simulink model "hybrid_lht_accumulator_backup"  (R2019b)
settings: Solver=FixedStepDiscrete  StartTime=0.0  StopTime=inf  FixedStep=1/bt.frequency  RelTol=1e-3
InitFcn:
  | ht_hybrid_setup;
StopFcn:
  | ht_hybrid_compare;
undefined symbols (not defined in the file or in its folder): bt, height, Ntheta, nTheta, width
libraries: hdlsllib x52, simulink x24, visionhdlutilities x2, dspsrcs4 x1, visionhdlio x1, lib_hybrid_ht_kernel x1, visionsources x1
(part 1 of 5)
settings Model: SimulationMode=accelerator  Creator=rgb11127  LastModifiedBy=rgb11127
settings DataIOCC: SaveOutput=off  SaveTime=off  ReturnWorkspaceOutputs=off

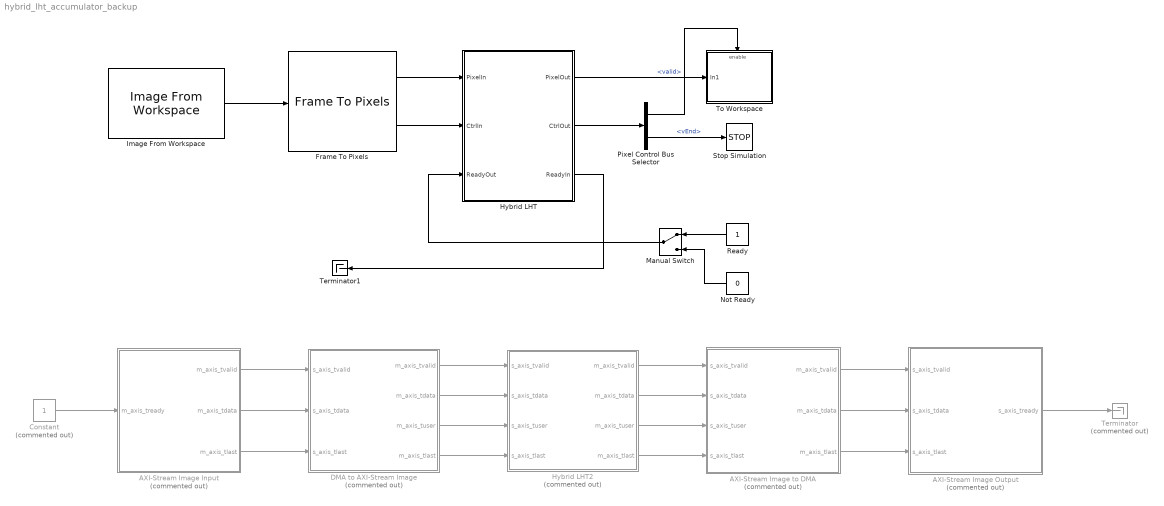
== system hybrid_lht_accumulator_backup ==
  AXI-Stream Image Input : Subsystem  Commented=on  mask{image=bt.inputImage, clk=1/150e6}
      mask prompts: image "Input Image:"; clk "Clock Rate:"
      mask init:
      | [height, width] = size(image);
      mask DialogControl DescGroupVar Prompt: AXI-Stream Image Input
      mask DialogControl DescTextVar Prompt: This block simulates an AXI-Stream image input for interfacing to a hardware accelerator or IP Core.
      mask DialogControl ParameterGroupVar Prompt: Main
  AXI-Stream Image Output : Subsystem  Commented=on  mask{height=bt.nRho, width=bt.nTheta, clk=1/150e6, d=0}
      mask prompts: height "Image Height:"; width "Image Width:"; clk "Clock Rate:"; d "Frame Capture Number"
      mask DialogControl DescGroupVar Prompt: AXI-Stream Image Output
      mask DialogControl DescTextVar Prompt: Image output using the AXI-Stream interface. Simulates an AXI DMA write channel.
      mask DialogControl ParameterGroupVar Prompt: Main
  AXI-Stream Image to DMA : Subsystem  Commented=on  mask{height=bt.nRho, width=bt.nTheta}
      mask prompts: height "Image Height"; width "Image Width"
      mask DialogControl DescGroupVar Prompt: AXI-Stream Image to DMA
      mask DialogControl DescTextVar Prompt: Converts from the AXI-Stream video standard to AXI-Stream DMA packet.
      mask DialogControl Container2 Prompt: Main
  Constant : Constant  Commented=on  OutDataTypeStr=boolean  SampleTime=-1
  DMA to AXI-Stream Image : Subsystem  Commented=on  mask{height=bt.height, width=bt.width}
      mask prompts: height "Image Height:"; width "Image Width:"
      mask DialogControl DescGroupVar Prompt: DMA to AXI-Stream Image
      mask DialogControl DescTextVar Prompt: Converts an DMA AXI-Stream packet to the AXI-Stream video standard.
      mask DialogControl Container2 Prompt: Main
  Frame To Pixels : visionhdlio/Frame To Pixels  NumComponents=1  NumPixels=1  VideoFormat=Custom  ActivePixelsPerLine=bt.width  ActiveVideoLines=bt.height  TotalPixelsPerLine=bt.widthpad  TotalVideoLines=bt.heightpad  StartingActiveLine=bt.activeline  FrontPorch=bt.frontporch  SampleTime=0
      settings: SourceProductName=Vision HDL Toolbox  SourceProductBaseCode=VT
  Hybrid LHT : Subsystem  TreatAsAtomicUnit=on
  Hybrid LHT2 : Subsystem  Commented=on
  Image From Workspace : visionsources/Image From Workspace  Tag=vipblks_nd  ImageValue=bt.inputImage  Ts=1/bt.fps  imagePorts=One multidimensional signal  OutPortLabels=R|G|B  ImageDataType=Inherit from 'Value'  Signed=on  WordLength=16  sdImageDataType=sfix(16)  FractionLengthMode=User-defined  FractionLength=15
      settings: SourceProductName=Computer Vision Toolbox  SourceProductBaseCode=VP
  Manual Switch : ManualSwitch
  Not Ready : Constant  Value=0  OutDataTypeStr=boolean  SampleTime=-1
  Pixel Control Bus Selector : BusSelector  OutputSignals=valid,vEnd
  Ready : Constant  OutDataTypeStr=boolean  SampleTime=-1
  Stop Simulation : Stop
  Terminator : Terminator  Commented=on
  Terminator1 : Terminator
  To Workspace : Subsystem  TreatAsAtomicUnit=on
  wires:
  Constant/1 -> AXI-Stream Image Input/1(m_axis_tready)
  AXI-Stream Image Input/1(m_axis_tvalid) -> DMA to AXI-Stream Image/1(s_axis_tvalid)
  AXI-Stream Image Input/2(m_axis_tdata) -> DMA to AXI-Stream Image/2(s_axis_tdata)
  AXI-Stream Image Input/3(m_axis_tlast) -> DMA to AXI-Stream Image/3(s_axis_tlast)
  DMA to AXI-Stream Image/1(m_axis_tvalid) -> Hybrid LHT2/1(s_axis_tvalid)
  DMA to AXI-Stream Image/2(m_axis_tdata) -> Hybrid LHT2/2(s_axis_tdata)
  DMA to AXI-Stream Image/3(m_axis_tuser) -> Hybrid LHT2/3(s_axis_tuser)
  DMA to AXI-Stream Image/4(m_axis_tlast) -> Hybrid LHT2/4(s_axis_tlast)
  AXI-Stream Image Output/1(s_axis_tready) -> Terminator/1
  AXI-Stream Image to DMA/3(m_axis_tlast) -> AXI-Stream Image Output/3(s_axis_tlast)
  AXI-Stream Image to DMA/2(m_axis_tdata) -> AXI-Stream Image Output/2(s_axis_tdata)
  AXI-Stream Image to DMA/1(m_axis_tvalid) -> AXI-Stream Image Output/1(s_axis_tvalid)
  Hybrid LHT2/4(m_axis_tlast) -> AXI-Stream Image to DMA/4(s_axis_tlast)
  Hybrid LHT2/3(m_axis_tuser) -> AXI-Stream Image to DMA/3(s_axis_tuser)
  Hybrid LHT2/2(m_axis_tdata) -> AXI-Stream Image to DMA/2(s_axis_tdata)
  Hybrid LHT2/1(m_axis_tvalid) -> AXI-Stream Image to DMA/1(s_axis_tvalid)
  Not Ready/1 -> Manual Switch/2
  Manual Switch/1 -> Hybrid LHT/3(ReadyOut)
  Ready/1 -> Manual Switch/1
  Hybrid LHT/3(ReadyIn) -> Terminator1/1
  Frame To Pixels/2 -> Hybrid LHT/2(CtrlIn)
  Frame To Pixels/1 -> Hybrid LHT/1(PixelIn)
  Hybrid LHT/2(CtrlOut) -> Pixel Control Bus Selector/1
  Hybrid LHT/1(PixelOut) -> To Workspace/1(In1)
  Pixel Control Bus Selector/1 -> To Workspace/Enable  "<valid>"
  Image From Workspace/1 -> Frame To Pixels/1
  Pixel Control Bus Selector/2 -> Stop Simulation/1  "<vEnd>"

== system hybrid_lht_accumulator_backup/AXI-Stream Image Input ==
  m_axis_tready : Inport
  Compare To Constant : simulink/Logic and Bit Operations/Compare To Constant  relop===  const=height*width-1  OutDataTypeStr=boolean
  HDL Counter : hdlsllib/Sources/HDL Counter  CountType=Count limited  CountInit=0  CountStep=1  CountMax=width*height-1  CountFromType=Initial value  CountFrom=0  CountResetPort=off  CountLoadPort=off  CountEnbPort=on  CountDirPort=off  CountDataType=Unsigned  CountWordLen=ceil(log2(width*height))  CountFracLen=0  CountSampTime=1
      settings: SourceProductName=Simulink
  Master AXI-Stream FIFO : Subsystem  mask{depth=32}
      mask prompts: depth "FIFO Depth:"
      mask DialogControl DescGroupVar Prompt: Master AXI-Stream FIFO
      mask DialogControl DescTextVar Prompt: A custom AXI-Stream FIFO for interfacing to write channel AXI DMAs.
      mask DialogControl ParameterGroupVar Prompt: Main
  Synchronous Image Source : Subsystem
  m_axis_tvalid : Outport
  m_axis_tdata : Outport  Port=2
  m_axis_tlast : Outport  Port=3
  wires:
  Master AXI-Stream FIFO/2(m_axis_tdata) -> m_axis_tdata/1
  Master AXI-Stream FIFO/3(m_axis_tlast) -> m_axis_tlast/1
  m_axis_tready/1 -> Master AXI-Stream FIFO/4(m_axis_tready)
  Master AXI-Stream FIFO/4(s_axis_tready) -> HDL Counter/1, Master AXI-Stream FIFO/1(s_axis_tvalid), Synchronous Image Source/Enable
  Compare To Constant/1 -> Master AXI-Stream FIFO/3(s_axis_tlast)
  Master AXI-Stream FIFO/1(m_axis_tvalid) -> m_axis_tvalid/1
  HDL Counter/1 -> Compare To Constant/1
  Synchronous Image Source/1(Pixel) -> Master AXI-Stream FIFO/2(s_axis_tdata)

== system hybrid_lht_accumulator_backup/AXI-Stream Image Output ==
  s_axis_tvalid : Inport
  s_axis_tdata : Inport  Port=2
  s_axis_tlast : Inport  Port=3
  AND1 : Logic  IconShape=distinctive  AllPortsSameDT=off  OutDataTypeStr=boolean
  Compare To Constant4 : simulink/Logic and Bit Operations/Compare To Constant  relop===  const=(height)*width-1  OutDataTypeStr=boolean
  Constant : Constant  OutDataTypeStr=boolean  SampleTime=-1
  Delay2 : Delay  DelayLength=d  ShowEnablePort=on
      settings: InputPortMap=u0,e6
  Pixel to Workspace : Subsystem
  Stop Simulation1 : Stop
  Terminator : Terminator
  Total Samples Counter : hdlsllib/Sources/HDL Counter  CountType=Count limited  CountInit=0  CountStep=1  CountMax=(height)*width-1  CountFromType=Initial value  CountFrom=0  CountResetPort=off  CountLoadPort=off  CountEnbPort=on  CountDirPort=off  CountDataType=Unsigned  CountWordLen=ceil(log2((height)*width+1))  CountFracLen=0  CountSampTime=1
      settings: SourceProductName=Simulink
  s_axis_tready : Outport  VectorParamsAs1DForOutWhenUnconnected=off
  wires:
  Constant/1 -> s_axis_tready/1, AND1/2
  s_axis_tlast/1 -> Terminator/1
  Delay2/1 -> Stop Simulation1/1
  Compare To Constant4/1 -> Delay2/1, Delay2/2
  Total Samples Counter/1 -> Compare To Constant4/1
  AND1/1 -> Pixel to Workspace/Enable, Total Samples Counter/1
  s_axis_tvalid/1 -> AND1/1
  s_axis_tdata/1 -> Pixel to Workspace/1(Pixel In)

== system hybrid_lht_accumulator_backup/AXI-Stream Image to DMA ==
  s_axis_tvalid : Inport
  s_axis_tdata : Inport  Port=2
  s_axis_tuser : Inport  Port=3
  s_axis_tlast : Inport  Port=4
  AND : Logic  IconShape=distinctive  AllPortsSameDT=off  OutDataTypeStr=boolean
  Compare To Constant : simulink/Logic and Bit Operations/Compare To Constant  relop===  const=height*width-1  OutDataTypeStr=boolean
  Data Type Conversion : DataTypeConversion  OutDataTypeStr=uint32
  Output Counter : hdlsllib/Sources/HDL Counter  CountType=Count limited  CountInit=0  CountStep=1  CountMax=height*width-1  CountFromType=Initial value  CountFrom=0  CountResetPort=off  CountLoadPort=off  CountEnbPort=on  CountDirPort=off  CountDataType=Unsigned  CountWordLen=ceil(log2(height*width))  CountFracLen=0  CountSampTime=1
      settings: SourceProductName=Simulink
  Terminator : Terminator
  Terminator1 : Terminator
  m_axis_tvalid : Outport
  m_axis_tdata : Outport  Port=2
  m_axis_tlast : Outport  Port=3
  wires:
  Data Type Conversion/1 -> m_axis_tdata/1
  s_axis_tdata/1 -> Data Type Conversion/1
  s_axis_tvalid/1 -> AND/2, m_axis_tvalid/1, Output Counter/1
  s_axis_tlast/1 -> Terminator/1
  s_axis_tuser/1 -> Terminator1/1
  Output Counter/1 -> Compare To Constant/1
  Compare To Constant/1 -> AND/1
  AND/1 -> m_axis_tlast/1

== system hybrid_lht_accumulator_backup/DMA to AXI-Stream Image ==
  s_axis_tvalid : Inport
  s_axis_tdata : Inport  Port=2
  s_axis_tlast : Inport  Port=3
  AND : Logic  IconShape=distinctive  AllPortsSameDT=off  OutDataTypeStr=boolean
  AND1 : Logic  IconShape=distinctive  AllPortsSameDT=off  OutDataTypeStr=boolean
  AND2 : Logic  IconShape=distinctive  AllPortsSameDT=off  OutDataTypeStr=boolean
  Compare To Constant : simulink/Logic and Bit Operations/Compare To Constant  relop===  const=width-1  OutDataTypeStr=boolean
  Compare To Zero : simulink/Logic and Bit Operations/Compare To Zero  relop===  OutDataTypeStr=boolean
  Compare To Zero1 : simulink/Logic and Bit Operations/Compare To Zero  relop===  OutDataTypeStr=boolean
  Terminator : Terminator
  X Counter : hdlsllib/Sources/HDL Counter  CountType=Count limited  CountInit=0  CountStep=1  CountMax=width-1  CountFromType=Initial value  CountFrom=0  CountResetPort=off  CountLoadPort=off  CountEnbPort=on  CountDirPort=off  CountDataType=Unsigned  CountWordLen=ceil(log2(width))  CountFracLen=0  CountSampTime=1
      settings: SourceProductName=Simulink
  Y Counter : hdlsllib/Sources/HDL Counter  CountType=Count limited  CountInit=0  CountStep=1  CountMax=height-1  CountFromType=Initial value  CountFrom=0  CountResetPort=off  CountLoadPort=off  CountEnbPort=on  CountDirPort=off  CountDataType=Unsigned  CountWordLen=ceil(log2(height))  CountFracLen=0  CountSampTime=1
      settings: SourceProductName=Simulink
  m_axis_tvalid : Outport
  m_axis_tdata : Outport  Port=2
  m_axis_tuser : Outport  Port=3
  m_axis_tlast : Outport  Port=4
  wires:
  AND2/1 -> m_axis_tlast/1
  Compare To Constant/1 -> Y Counter/1, AND2/2
  AND1/1 -> m_axis_tuser/1
  AND/1 -> AND1/2
  s_axis_tlast/1 -> Terminator/1
  Compare To Zero/1 -> AND/2
  Compare To Zero1/1 -> AND/1
  Y Counter/1 -> Compare To Zero/1
  X Counter/1 -> Compare To Constant/1, Compare To Zero1/1
  s_axis_tvalid/1 -> m_axis_tvalid/1, AND1/1, AND2/1, X Counter/1
  s_axis_tdata/1 -> m_axis_tdata/1

== system hybrid_lht_accumulator_backup/Hybrid LHT ==
  PixelIn : Inport
  CtrlIn : Inport  Port=2
  ReadyOut : Inport  Port=3
  Constant : Constant  Value=60  OutDataTypeStr=uint32  SampleTime=-1
  FIFO Subsystem : Subsystem
  Hybrid LHT Accumulator : Subsystem  AncestorBlock=lib_hybrid_ht_accumulator/Hybrid LHT Accumulator  VariantControl=Basic  mask{w=bt.width, h=bt.height, theta=bt.theta, mode=Parameter Space Readout}
      mask prompts: w "Image Width:"; h "Image Height:"; theta "Orientations:"; mode "Architecture:"
      mask init:
      | % Get parameters
      | maxRho = ceil(sqrt((h/2)^2+(w/2)^2));
      | Nrho = maxRho*2;
      | [~, Ntheta] = size(theta);
      | 
      | % Set correct variants
      | 
      | blk_gen = [gcb, '/Simple Hough Accumulator/Flag Generator'];
      | blk_sep = [gcb, '/Simple Hough Accumulator/Separate Bits'];
      | blk_keep = [gcb, '/Simple Hough Accumulator/Keep Flag'];
      | blk_out = [gcb, '/Output Generation'];
      | 
      | oldVariant = get_param(blk_gen, 'OverrideUsingVariant');
      | 
      | switch get_param(gcb, 'mode')
      |     case 'Video Backprojection'
      |         newVariant = 'Backprojection';
      |         voteWL = ceil(log2(2*maxRho))+1;
      |         videomode = 1;
      |     case 'Parameter Space Readout'
      |         newVariant = 'Passthrough';
      |         voteWL = ceil(log2(2*maxRho));
      |         videomode = 0;
      |     otherwise
      |         newVariant = 'Passthrough';
      |         voteWL = ceil(log2(2*maxRho));
      |         videomode = 0;
      | end
      | 
      | if ~strcmp(oldVariant, newVariant)
      |     set_param(blk_gen, 'OverrideUsingVariant', newVariant);
      |     set_param(blk_sep, 'OverrideUsingVariant', newVariant);
      |     set_param(blk_keep, 'OverrideUsingVariant', newVariant);
      |     set_param(blk_out, 'OverrideUsingVariant', newVariant);
      | end
      mask TypeOptions mode: Video Backprojection | Parameter Space Readout
      mask DialogControl DescGroupVar Prompt: Parallel Hough Accumulator
      mask DialogControl DescTextVar Prompt: The Parallel Hough Accumulator implements a low-latency circuit for storing the Hough Parameter Space. If the mode input is set to '1', the architecture will draw lines using backpropagation. If mode is set to '0', the HPS is output on the HPS and CtrlOut ports.
      mask DialogControl Container2 Prompt: Image Parameters
      mask DialogControl Container3 Prompt: Accumulator Implementation
  Hybrid LHT Kernel : lib_hybrid_ht_kernel/Hybrid LHT Kernel  w=bt.width  h=bt.height  theta=bt.theta
  NOT : Logic  Operator=NOT  IconShape=distinctive  AllPortsSameDT=off  OutDataTypeStr=boolean
  PixelOut : Outport  VectorParamsAs1DForOutWhenUnconnected=off
  CtrlOut : Outport  Port=2  VectorParamsAs1DForOutWhenUnconnected=off
  ReadyIn : Outport  Port=3  VectorParamsAs1DForOutWhenUnconnected=off
  wires:
  NOT/1 -> ReadyIn/1
  ReadyOut/1 -> Hybrid LHT Accumulator/6(Ready)
  FIFO Subsystem/3(ReadyIn) -> NOT/1
  Hybrid LHT Accumulator/2(CtrlOut) -> CtrlOut/1
  PixelIn/1 -> FIFO Subsystem/1(PixelIn)
  CtrlIn/1 -> FIFO Subsystem/2(CtrlIn)
  Hybrid LHT Kernel/2 -> Hybrid LHT Accumulator/3(Rho)
  Hybrid LHT Kernel/3 -> Hybrid LHT Accumulator/4(Shift)
  FIFO Subsystem/2(CtrlOut) -> Hybrid LHT Kernel/2
  Hybrid LHT Kernel/5 -> FIFO Subsystem/3(POP)
  Hybrid LHT Kernel/1 -> Hybrid LHT Accumulator/2(vEdge)
  Constant/1 -> Hybrid LHT Accumulator/1(Threshold)
  FIFO Subsystem/1(PixelOut) -> Hybrid LHT Kernel/1
  Hybrid LHT Kernel/4 -> Hybrid LHT Accumulator/5(CtrlIn)
  Hybrid LHT Accumulator/1(Pixel) -> PixelOut/1

== system hybrid_lht_accumulator_backup/Hybrid LHT2 ==
  s_axis_tvalid : Inport
  s_axis_tdata : Inport  Port=2
  s_axis_tuser : Inport  Port=3
  s_axis_tlast : Inport  Port=4
  Constant : Constant  Commented=on  OutDataTypeStr=uint8  SampleTime=-1
  Constant1 : Constant  Commented=on  OutDataTypeStr=boolean  SampleTime=-1
  Hybrid LHT Accumulator : Subsystem  mask{height=bt.height, width=bt.width, theta=bt.theta}
      mask prompts: height "Image Height:"; width "Image Width:"; theta "Orientations:"
      mask init:
      | maxRho = ceil(sqrt((height/2)^2+(width/2)^2));
      | nRho = maxRho*2;
      | [~, nTheta] = size(theta);
      | 
      | voteWL = ceil(log2(2*maxRho));
      mask DialogControl ParameterGroupVar Prompt: Main
  Hybrid LHT Accumulator2 : Subsystem  Commented=on  VariantControl=Basic  mask{w=bt.width, h=bt.height, theta=bt.theta, mode=Parameter Space Readout}
      mask prompts: w "Image Width:"; h "Image Height:"; theta "Orientations:"; mode "Architecture:"
      mask init: same as hybrid_lht_accumulator_backup/Hybrid LHT/Hybrid LHT Accumulator
      mask TypeOptions mode: Video Backprojection | Parameter Space Readout
      mask DialogControl DescGroupVar Prompt: Parallel Hough Accumulator
      mask DialogControl DescTextVar Prompt: The Parallel Hough Accumulator implements a low-latency circuit for storing the Hough Parameter Space. If the mode input is set to '1', the architecture will draw lines using backpropagation. If mode is set to '0', the HPS is output on the HPS and CtrlOut ports.
      mask DialogControl Container2 Prompt: Image Parameters
      mask DialogControl Container3 Prompt: Accumulator Implementation
  Hybrid LHT Kernel : Subsystem  mask{height=bt.height, width=bt.width, theta=bt.theta}
      mask prompts: height "Image Height:"; width "Image Width:"; theta "Orientations:"
      mask init:
      | % Get number of orientations to operate across
      | [~, nTheta] = size(theta);
      | 
      | % Get discretisation step of theta
      | if nTheta > 1
      |     dTheta = theta(end) - theta(end-1);
      | else
      |     dTheta = 1;
      | end
      | 
      | % Get the maximum magnitude of displacement
      | maxRho = ceil(sqrt((height/2)^2+(width/2)^2));
      | 
      | % Get the number of bits required to vote correctly
      | voteWL = ceil(log2(maxRho*2));
      | 
      | % Get the number of division possible
      | if nTheta < floor(36/voteWL)
      |     L = nTheta;
      | else
      |     L = floor(36/voteWL);
      | end
      | 
      | % Set lambda, the number of orientations to operate across per gradient
      | % orientation given
      | lambda = floor(nTheta/(2*L));
      | 
      | % Determine if the number of orientations is odd. This will prevent over
      | % use of the parameter space.
      | if lambda == 0
      |     subflag = 0;
      | else
      |     subflag = ~mod(nTheta/(L), 2);
      | end
      | 
      | % Get the limits so that we can determine the number of bits to shift
      | % the votes
      | U = floor(nTheta/L):floor(nTheta/L):nTheta;
      | D = 0:floor(nTheta/L):nTheta-1;
      mask DialogControl ParameterGroupVar Prompt: Main
  Hybrid LHT Kernel1 : Subsystem  Commented=on  mask{height=bt.height, width=bt.width, theta=bt.theta}
      mask prompts: height "Image Height:"; width "Image Width:"; theta "Orientations:"
      mask init: same as hybrid_lht_accumulator_backup/Hybrid LHT2/Hybrid LHT Kernel
      mask DialogControl ParameterGroupVar Prompt: Main
  Hybrid LHT Kernel2 : Subsystem  Commented=on  mask{w=bt.width, h=bt.height, theta=bt.theta}
      mask prompts: w "Image Width:"; h "Image Height:"; theta "Orientations:"
      mask init:
      | % Get number of orientations to operate across
      | [~, Ntheta] = size(theta);
      | 
      | % Get discretisation step of theta
      | if Ntheta > 1
      |     dTheta = theta(end) - theta(end-1);
      | else
      |     dTheta = 1;
      | end
      | 
      | % Get the maximum magnitude of displacement
      | maxRho = ceil(sqrt((h/2)^2+(w/2)^2));
      | 
      | % Get the number of bits required to vote correctly
      | voteWL = ceil(log2(maxRho*2));
      | 
      | % Get the number of division possible
      | if Ntheta < floor(36/voteWL)
      |     L = Ntheta;
      | else
      |     L = floor(36/voteWL);
      | end
      | 
      | % Set lambda, the number of orientations to operate across per gradient
      | % orientation given
      | lambda = floor(Ntheta/(2*L));
      | 
      | % Determine if the number of orientations is odd. This will prevent over
      | % use of the parameter space.
      | if lambda == 0
      |     subflag = 0;
      | else
      |     subflag = ~mod(floor(Ntheta/(L)), 2);
      | end
      | 
      | % Get the limits so that we can determine the number of bits to shift
      | % the votes
      | U = floor(Ntheta/L):floor(Ntheta/L):Ntheta-floor(Ntheta/L);
      | D = 0:floor(Ntheta/L):Ntheta-1;
      mask DialogControl DescGroupVar Prompt: Parallel LHT Kernel
      mask DialogControl DescTextVar Prompt: This block implements a Parallel Hough Kernel for the Line Hough Transform. A Symmetric Kernel can be selected that reduces the DSP consumption. The symmetric architecture can only be selected if there are an even number of orientation values (more than 2), and the orientation values are symmetric about 90 degrees.
      mask DialogControl ParameterGroupVar Prompt: Image Parameters
      mask DialogControl Container3 Prompt: Hough Kernel Implementation
  m_axis_tvalid : Outport
  m_axis_tdata : Outport  Port=2
  m_axis_tuser : Outport  Port=3
  m_axis_tlast : Outport  Port=4
  wires:
  Constant/1 -> Hybrid LHT Accumulator2/1(Threshold)
  Constant1/1 -> Hybrid LHT Accumulator2/6(Ready)
  Hybrid LHT Kernel2/1(vEdge) -> Hybrid LHT Accumulator2/2(vEdge)
  Hybrid LHT Kernel2/2(Rho) -> Hybrid LHT Accumulator2/3(Rho)
  Hybrid LHT Kernel2/3(Shift) -> Hybrid LHT Accumulator2/4(Shift)
  Hybrid LHT Kernel2/4(valid_out) -> Hybrid LHT Accumulator2/7(valid_in)
  Hybrid LHT Kernel2/5(user_out) -> Hybrid LHT Accumulator2/8(user_in)
  Hybrid LHT Kernel2/6(last_out) -> Hybrid LHT Accumulator2/5(last_in)
  Hybrid LHT Kernel/1(m_axis_tvalid) -> Hybrid LHT Accumulator/1(s_axis_tvalid)
  Hybrid LHT Kernel/2(m_axis_tuser) -> Hybrid LHT Accumulator/2(s_axis_tuser)
  Hybrid LHT Kernel/3(m_axis_tlast) -> Hybrid LHT Accumulator/3(s_axis_tlast)
  Hybrid LHT Kernel/4(hough_param) -> Hybrid LHT Accumulator/4(hough_param)
  Hybrid LHT Kernel/5(edge) -> Hybrid LHT Accumulator/5(edge)
  Hybrid LHT Kernel/6(shift) -> Hybrid LHT Accumulator/6(shift)
  Hybrid LHT Accumulator/1(m_axis_tvalid) -> m_axis_tvalid/1
  Hybrid LHT Accumulator/2(m_axis_tdata) -> m_axis_tdata/1
  Hybrid LHT Accumulator/3(m_axis_tuser) -> m_axis_tuser/1
  Hybrid LHT Accumulator/4(m_axis_tlast) -> m_axis_tlast/1
  s_axis_tvalid/1 -> Hybrid LHT Kernel/1(s_axis_tvalid)
  s_axis_tdata/1 -> Hybrid LHT Kernel/2(s_axis_tdata)
  s_axis_tuser/1 -> Hybrid LHT Kernel/3(s_axis_tuser)
  s_axis_tlast/1 -> Hybrid LHT Kernel/4(s_axis_tlast)

== system hybrid_lht_accumulator_backup/To Workspace ==
  In1 : Inport
  Enable : EnablePort
  To Workspace : ToWorkspace  VariableName=dataout  SampleTime=-1
      settings: Save2DSignal=2-D array (concatenate along first dimension)
  wires:
  In1/1 -> To Workspace/1

== system hybrid_lht_accumulator_backup/AXI-Stream Image Input/Master AXI-Stream FIFO ==
  s_axis_tvalid : Inport
  s_axis_tdata : Inport  Port=2
  s_axis_tlast : Inport  Port=3
  m_axis_tready : Inport  Port=4
  AND : Logic  IconShape=distinctive  AllPortsSameDT=off  OutDataTypeStr=boolean
  "Compare To Constant " : simulink/Logic and Bit Operations/Compare To Constant  relop=>=  const=floor(depth/2)  OutDataTypeStr=boolean
  Delay : Delay  DelayLength=1
  HDL FIFO TDATA : hdlsllib/HDL RAMs/HDL FIFO  fifo_size=depth  mode=Classic  ratio=1  push_msg=Error  pop_msg=Error  show_empty=on  show_full=off  show_num=on  LabelModeActiveChoice_Mode=Classic
      settings: SourceProductName=Simulink  SourceProductBaseCode=SL
  HDL FIFO TLAST : hdlsllib/HDL RAMs/HDL FIFO  fifo_size=depth  mode=Classic  ratio=1  push_msg=Error  pop_msg=Error  show_empty=off  show_full=off  show_num=off  LabelModeActiveChoice_Mode=Classic
      settings: SourceProductName=Simulink  SourceProductBaseCode=SL
  NOT : Logic  Operator=NOT  IconShape=distinctive  AllPortsSameDT=off  OutDataTypeStr=boolean
  NOT1 : Logic  Operator=NOT  IconShape=distinctive  AllPortsSameDT=off  OutDataTypeStr=boolean
  m_axis_tvalid : Outport  VectorParamsAs1DForOutWhenUnconnected=off
  m_axis_tdata : Outport  Port=2  VectorParamsAs1DForOutWhenUnconnected=off
  m_axis_tlast : Outport  Port=3  VectorParamsAs1DForOutWhenUnconnected=off
  s_axis_tready : Outport  Port=4
  wires:
  Delay/1 -> m_axis_tvalid/1
  s_axis_tvalid/1 -> HDL FIFO TDATA/2, HDL FIFO TLAST/2
  s_axis_tdata/1 -> HDL FIFO TDATA/1
  s_axis_tlast/1 -> HDL FIFO TLAST/1
  "Compare To Constant "/1 -> NOT1/1
  NOT1/1 -> s_axis_tready/1
  HDL FIFO TDATA/3 -> "Compare To Constant "/1
  m_axis_tready/1 -> AND/1
  NOT/1 -> AND/2, Delay/1
  AND/1 -> HDL FIFO TDATA/3, HDL FIFO TLAST/3
  HDL FIFO TDATA/2 -> NOT/1
  HDL FIFO TLAST/1 -> m_axis_tlast/1
  HDL FIFO TDATA/1 -> m_axis_tdata/1

== system hybrid_lht_accumulator_backup/AXI-Stream Image Input/Synchronous Image Source ==
  Enable : EnablePort
  Signal From Workspace : dspsrcs4/Signal From Workspace  X=reshape((image)', [height*width, 1])  Ts=clk  nsamps=1  OutputAfterFinalValue=Cyclic repetition  ignoreOrWarnInputAndFrameLengths=off  OutputFrames=off
  Pixel : Outport
  wires:
  Signal From Workspace/1 -> Pixel/1

== system hybrid_lht_accumulator_backup/AXI-Stream Image Output/Pixel to Workspace ==
  Pixel In : Inport
  Enable : EnablePort
  To Workspace : ToWorkspace  VariableName=simout  SampleTime=-1
      settings: MaxDataPoints=height*width  Save2DSignal=2-D array (concatenate along first dimension)
  wires:
  Pixel In/1 -> To Workspace/1

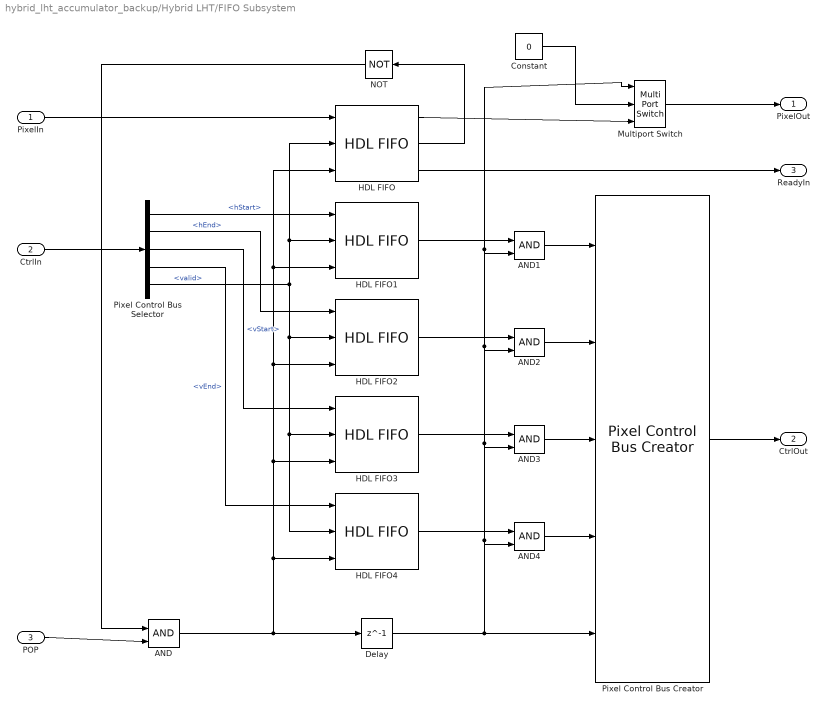
== system hybrid_lht_accumulator_backup/Hybrid LHT/FIFO Subsystem ==
  PixelIn : Inport
  CtrlIn : Inport  Port=2
  POP : Inport  Port=3
  AND{,1..4} (5 alike) : Logic  IconShape=distinctive  AllPortsSameDT=off  OutDataTypeStr=boolean
  Constant : Constant  Value=0  OutDataTypeStr=fixdt(0, 9, 0)  SampleTime=-1
  Delay : Delay  DelayLength=1
  HDL FIFO : hdlsllib/HDL RAMs/HDL FIFO  fifo_size=512  mode=Classic  ratio=1  push_msg=Warning  pop_msg=Warning  show_empty=on  show_full=on  show_num=off  LabelModeActiveChoice_Mode=Classic
      settings: SourceProductName=HDL Coder  SourceProductBaseCode=HD
  HDL FIFO{1..4} (4 alike) : hdlsllib/HDL RAMs/HDL FIFO  fifo_size=512  mode=Classic  ratio=1  push_msg=Warning  pop_msg=Warning  show_empty=off  show_full=off  show_num=off  LabelModeActiveChoice_Mode=Classic
      settings: SourceProductName=HDL Coder  SourceProductBaseCode=HD
  Multiport Switch : MultiPortSwitch  DataPortOrder=Zero-based contiguous  Inputs=2  zeroidx=on
  NOT : Logic  Operator=NOT  IconShape=distinctive  AllPortsSameDT=off  OutDataTypeStr=boolean
  Pixel Control Bus Creator : visionhdlutilities/Pixel Control Bus Creator
      settings: SourceProductName=Vision HDL Toolbox  SourceProductBaseCode=VT
  Pixel Control Bus Selector : BusSelector  OutputSignals=hStart,hEnd,vStart,vEnd,valid
  PixelOut : Outport  VectorParamsAs1DForOutWhenUnconnected=off
  CtrlOut : Outport  Port=2  VectorParamsAs1DForOutWhenUnconnected=off
  ReadyIn : Outport  Port=3  VectorParamsAs1DForOutWhenUnconnected=off
  wires:
  AND4/1 -> Pixel Control Bus Creator/4
  HDL FIFO4/1 -> AND4/1
  AND3/1 -> Pixel Control Bus Creator/3
  HDL FIFO3/1 -> AND3/1
  AND2/1 -> Pixel Control Bus Creator/2
  HDL FIFO2/1 -> AND2/1
  AND1/1 -> Pixel Control Bus Creator/1
  HDL FIFO1/1 -> AND1/1
  NOT/1 -> AND/1
  HDL FIFO/2 -> NOT/1
  AND/1 -> Delay/1, HDL FIFO4/3, HDL FIFO3/3, HDL FIFO1/3, HDL FIFO/3, HDL FIFO2/3
  POP/1 -> AND/2
  HDL FIFO/3 -> ReadyIn/1
  Pixel Control Bus Selector/4 -> HDL FIFO4/1  "<vEnd>"
  Pixel Control Bus Selector/3 -> HDL FIFO3/1  "<vStart>"
  Pixel Control Bus Selector/2 -> HDL FIFO2/1  "<hEnd>"
  Pixel Control Bus Selector/5 -> HDL FIFO1/2, HDL FIFO/2, HDL FIFO2/2, HDL FIFO3/2, HDL FIFO4/2  "<valid>"
  Pixel Control Bus Creator/1 -> CtrlOut/1
  Pixel Control Bus Selector/1 -> HDL FIFO1/1  "<hStart>"
  CtrlIn/1 -> Pixel Control Bus Selector/1
  PixelIn/1 -> HDL FIFO/1
  Multiport Switch/1 -> PixelOut/1
  HDL FIFO/1 -> Multiport Switch/3
  Delay/1 -> Pixel Control Bus Creator/5, Multiport Switch/1, AND1/2, AND2/2, AND3/2, AND4/2
  Constant/1 -> Multiport Switch/2

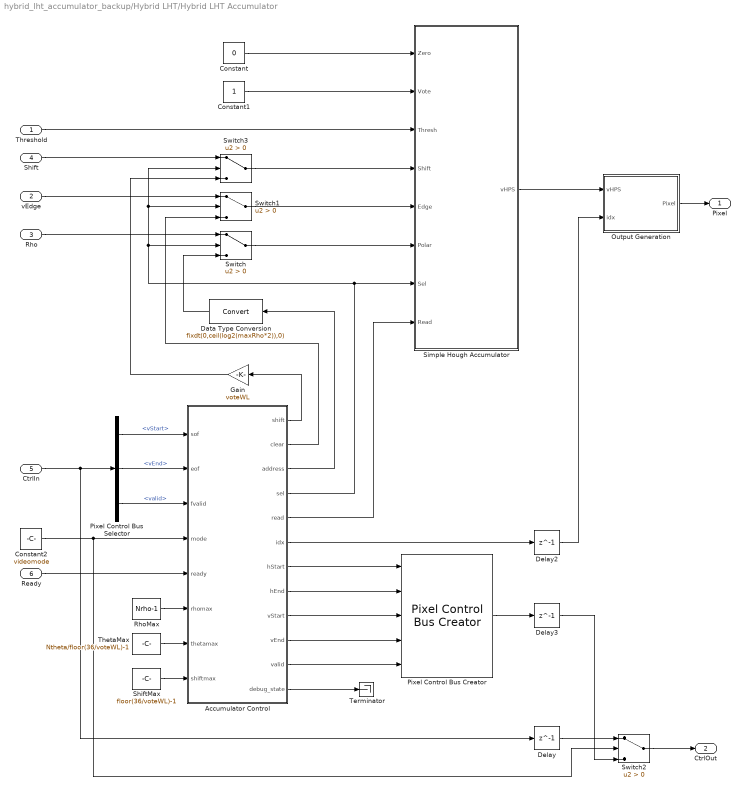
== system hybrid_lht_accumulator_backup/Hybrid LHT/Hybrid LHT Accumulator ==
  Threshold : Inport
  vEdge : Inport  Port=2
  Rho : Inport  Port=3
  Shift : Inport  Port=4
  CtrlIn : Inport  Port=5
  Ready : Inport  Port=6
  Accumulator Control : MATLAB Function  TreatAsAtomicUnit=on
  Constant : Constant  Value=0  OutDataTypeStr=fixdt(0,ceil(log2(maxRho*2)),0)  SampleTime=-1
  Constant1 : Constant  OutDataTypeStr=fixdt(0,ceil(log2(maxRho*2)),0)  SampleTime=-1
  Constant2 : Constant  Value=videomode  OutDataTypeStr=boolean  SampleTime=-1
  Data Type Conversion : DataTypeConversion  OutDataTypeStr=fixdt(0,ceil(log2(maxRho*2)),0)  RndMeth=Round
  Delay : Delay  DelayLength=1
  Delay2 : Delay  DelayLength=1
  Delay3 : Delay  DelayLength=1
  Gain : Gain  Gain=voteWL  OutDataTypeStr=fixdt(0, 6, 0)
  Output Generation : Subsystem  VariantControlMode=Label  Variant=on  VariantControl=Variant1  LabelModeActiveChoice=Passthrough
  Pixel Control Bus Selector : BusSelector  OutputSignals=vStart,vEnd,valid
  Pixel Control Bus Creator : visionhdlutilities/Pixel Control Bus Creator
      settings: SourceProductName=Vision HDL Toolbox  SourceProductBaseCode=VT
  RhoMax : Constant  Value=Nrho-1  OutDataTypeStr=uint32  SampleTime=-1
  ShiftMax : Constant  Value=floor(36/voteWL)-1  OutDataTypeStr=fixdt(0, floor(36/voteWL), 0)  SampleTime=-1
  Simple Hough Accumulator : Subsystem
  Switch{,1..3} (4 alike) : Switch  Criteria=u2 > Threshold
  Terminator : Terminator
  ThetaMax : Constant  Value=Ntheta/floor(36/voteWL)-1  OutDataTypeStr=uint32  SampleTime=-1
  Pixel : Outport  VectorParamsAs1DForOutWhenUnconnected=off
  CtrlOut : Outport  Port=2  VectorParamsAs1DForOutWhenUnconnected=off
  wires:
  Ready/1 -> Accumulator Control/5(ready)
  Constant/1 -> Simple Hough Accumulator/1(Zero)
  Constant1/1 -> Simple Hough Accumulator/2(Vote)
  Switch/1 -> Simple Hough Accumulator/6(Polar)
  CtrlIn/1 -> Pixel Control Bus Selector/1, Delay/1
  Pixel Control Bus Selector/3 -> Accumulator Control/3(fvalid)  "<valid>"
  Pixel Control Bus Selector/2 -> Accumulator Control/2(eof)  "<vEnd>"
  Pixel Control Bus Selector/1 -> Accumulator Control/1(sof)  "<vStart>"
  Accumulator Control/7(hStart) -> Pixel Control Bus Creator/1
  Accumulator Control/8(hEnd) -> Pixel Control Bus Creator/2
  Accumulator Control/9(vStart) -> Pixel Control Bus Creator/3
  Accumulator Control/10(vEnd) -> Pixel Control Bus Creator/4
  Accumulator Control/11(valid) -> Pixel Control Bus Creator/5
  Accumulator Control/4(sel) -> Switch/2, Switch3/2, Switch1/2, Simple Hough Accumulator/7(Sel)
  Switch1/1 -> Simple Hough Accumulator/5(Edge)
  Accumulator Control/6(idx) -> Delay2/1
  Threshold/1 -> Simple Hough Accumulator/3(Thresh)
  Accumulator Control/5(read) -> Simple Hough Accumulator/8(Read)
  RhoMax/1 -> Accumulator Control/6(rhomax)
  ThetaMax/1 -> Accumulator Control/7(thetamax)
  Pixel Control Bus Creator/1 -> Delay3/1
  Switch2/1 -> CtrlOut/1
  Constant2/1 -> Accumulator Control/4(mode), Switch2/2
  Rho/1 -> Switch/1
  Accumulator Control/3(address) -> Data Type Conversion/1
  Output Generation/1(" Pixel") -> Pixel/1
  Delay3/1 -> Switch2/3
  Delay/1 -> Switch2/1
  Delay2/1 -> Output Generation/2("idx ")
  Accumulator Control/2(clear) -> Switch1/3
  Data Type Conversion/1 -> Switch/3
  Accumulator Control/12(debug_state) -> Terminator/1
  Shift/1 -> Switch3/1
  ShiftMax/1 -> Accumulator Control/8(shiftmax)
  Accumulator Control/1(shift) -> Gain/1
  Switch3/1 -> Simple Hough Accumulator/4(Shift)
  Gain/1 -> Switch3/3
  Simple Hough Accumulator/1(vHPS) -> Output Generation/1("vHPS ")
  vEdge/1 -> Switch1/1

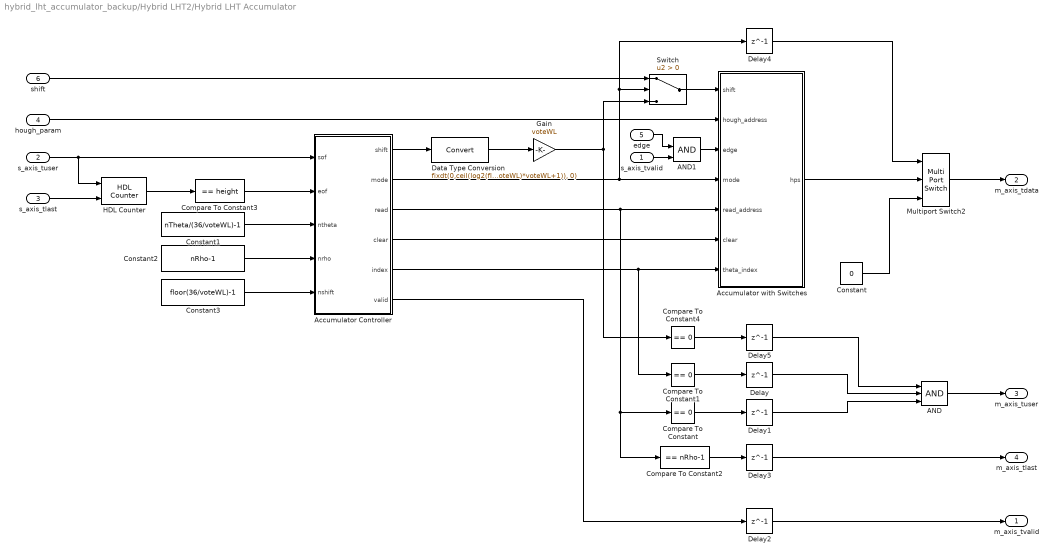
== system hybrid_lht_accumulator_backup/Hybrid LHT2/Hybrid LHT Accumulator ==
  s_axis_tvalid : Inport
  s_axis_tuser : Inport  Port=2
  s_axis_tlast : Inport  Port=3
  hough_param : Inport  Port=4
  edge : Inport  Port=5
  shift : Inport  Port=6
  AND : Logic  Inputs=3  IconShape=distinctive  AllPortsSameDT=off  OutDataTypeStr=boolean
  AND1 : Logic  IconShape=distinctive  AllPortsSameDT=off  OutDataTypeStr=boolean
  Accumulator Controller : MATLAB Function  TreatAsAtomicUnit=on
  Accumulator with Switches : Subsystem
  Compare To Constant : simulink/Logic and Bit Operations/Compare To Constant  relop===  const=0  OutDataTypeStr=boolean
  Compare To Constant1 : simulink/Logic and Bit Operations/Compare To Constant  relop===  const=0  OutDataTypeStr=boolean
  Compare To Constant2 : simulink/Logic and Bit Operations/Compare To Constant  relop===  const=nRho-1  OutDataTypeStr=boolean
  Compare To Constant3 : simulink/Logic and Bit Operations/Compare To Constant  relop===  const=height  OutDataTypeStr=boolean
  Compare To Constant4 : simulink/Logic and Bit Operations/Compare To Constant  relop===  const=0  OutDataTypeStr=boolean
  Constant : Constant  Value=0  OutDataTypeStr=fixdt(0, ceil(log2(2*maxRho)), 0)  SampleTime=-1
  Constant1 : Constant  Value=nTheta/(36/voteWL)-1  OutDataTypeStr=uint16  SampleTime=-1
  Constant2 : Constant  Value=nRho-1  OutDataTypeStr=uint16  SampleTime=-1
  Constant3 : Constant  Value=floor(36/voteWL)-1  OutDataTypeStr=fixdt(0, floor(36/voteWL), 0)  SampleTime=-1
  Data Type Conversion : DataTypeConversion  OutDataTypeStr=fixdt(0,ceil(log2(floor(36/voteWL)*voteWL+1)), 0)
  Delay{,1..5} (6 alike) : Delay  DelayLength=1
  Gain : Gain  Gain=voteWL  OutDataTypeStr=fixdt(0,ceil(log2(floor(36/voteWL)*voteWL+1)), 0)
  HDL Counter : hdlsllib/Sources/HDL Counter  CountType=Count limited  CountInit=0  CountStep=1  CountMax=height  CountFromType=Initial value  CountFrom=0  CountResetPort=on  CountLoadPort=off  CountEnbPort=on  CountDirPort=off  CountDataType=Unsigned  CountWordLen=ceil(log2(height+1))  CountFracLen=0  CountSampTime=1
      settings: SourceProductName=Simulink
  Multiport Switch2 : MultiPortSwitch  DataPortOrder=Zero-based contiguous  Inputs=2  zeroidx=on
  Switch : Switch  Criteria=u2 > Threshold
  m_axis_tvalid : Outport
  m_axis_tdata : Outport  Port=2
  m_axis_tuser : Outport  Port=3
  m_axis_tlast : Outport  Port=4
  wires:
  s_axis_tvalid/1 -> AND1/2
  AND1/1 -> Accumulator with Switches/3(edge)
  edge/1 -> AND1/1
  Data Type Conversion/1 -> Gain/1
  Gain/1 -> Compare To Constant4/1, Switch/3
  Constant3/1 -> Accumulator Controller/5(nshift)
  Delay/1 -> AND/2
  Delay1/1 -> AND/3
  Compare To Constant4/1 -> Delay5/1
  Delay5/1 -> AND/1
  Accumulator Controller/1(shift) -> Data Type Conversion/1
  shift/1 -> Switch/1
  Switch/1 -> Accumulator with Switches/1(shift)
  Accumulator Controller/4(clear) -> Accumulator with Switches/6(clear)
  Accumulator Controller/2(mode) -> Delay4/1, Switch/2, Accumulator with Switches/4(mode)
  Accumulator Controller/3(read) -> Accumulator with Switches/5(read_address), Compare To Constant2/1, Compare To Constant/1
  Constant1/1 -> Accumulator Controller/3(ntheta)
  Accumulator Controller/5(index) -> Compare To Constant1/1, Accumulator with Switches/7(theta_index)
  Compare To Constant2/1 -> Delay3/1
  Constant2/1 -> Accumulator Controller/4(nrho)
  s_axis_tuser/1 -> Accumulator Controller/1(sof), HDL Counter/1
  Compare To Constant1/1 -> Delay/1
  Compare To Constant/1 -> Delay1/1
  Delay3/1 -> m_axis_tlast/1
  hough_param/1 -> Accumulator with Switches/2(hough_address)
  AND/1 -> m_axis_tuser/1
  HDL Counter/1 -> Compare To Constant3/1
  s_axis_tlast/1 -> HDL Counter/2
  Compare To Constant3/1 -> Accumulator Controller/2(eof)
  Multiport Switch2/1 -> m_axis_tdata/1
  Accumulator with Switches/1(hps) -> Multiport Switch2/2
  Constant/1 -> Multiport Switch2/3
  Accumulator Controller/6(valid) -> Delay2/1
  Delay2/1 -> m_axis_tvalid/1
  Delay4/1 -> Multiport Switch2/1

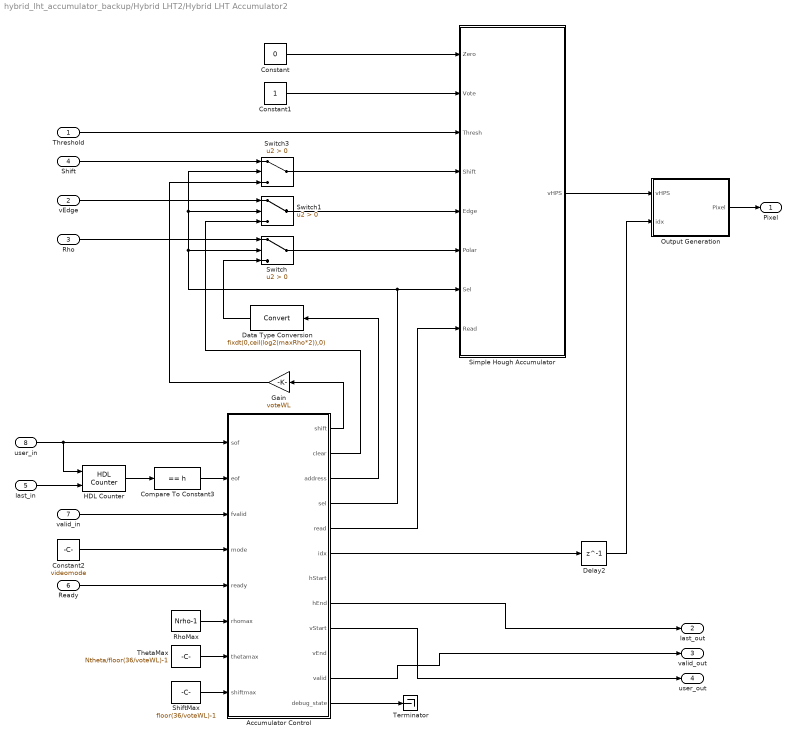
== system hybrid_lht_accumulator_backup/Hybrid LHT2/Hybrid LHT Accumulator2 ==
  Threshold : Inport
  vEdge : Inport  Port=2
  Rho : Inport  Port=3
  Shift : Inport  Port=4
  last_in : Inport  Port=5
  Ready : Inport  Port=6
  valid_in : Inport  Port=7
  user_in : Inport  Port=8
  Accumulator Control : MATLAB Function  TreatAsAtomicUnit=on
  Compare To Constant3 : simulink/Logic and Bit Operations/Compare To Constant  relop===  const=h  OutDataTypeStr=boolean
  Constant : Constant  Value=0  OutDataTypeStr=fixdt(0,ceil(log2(maxRho*2)),0)  SampleTime=-1
  Constant1 : Constant  OutDataTypeStr=fixdt(0,ceil(log2(maxRho*2)),0)  SampleTime=-1
  Constant2 : Constant  Value=videomode  OutDataTypeStr=boolean  SampleTime=-1
  Data Type Conversion : DataTypeConversion  OutDataTypeStr=fixdt(0,ceil(log2(maxRho*2)),0)  RndMeth=Round
  Delay2 : Delay  DelayLength=1
  Gain : Gain  Gain=voteWL  OutDataTypeStr=fixdt(0, 6, 0)
  HDL Counter : hdlsllib/Sources/HDL Counter  CountType=Count limited  CountInit=0  CountStep=1  CountMax=h  CountFromType=Initial value  CountFrom=0  CountResetPort=on  CountLoadPort=off  CountEnbPort=on  CountDirPort=off  CountDataType=Unsigned  CountWordLen=ceil(log2(h+1))  CountFracLen=0  CountSampTime=1
      settings: SourceProductName=Simulink
  Output Generation : Subsystem  VariantControlMode=Label  Variant=on  VariantControl=Variant1  LabelModeActiveChoice=Passthrough
  RhoMax : Constant  Value=Nrho-1  OutDataTypeStr=uint32  SampleTime=-1
  ShiftMax : Constant  Value=floor(36/voteWL)-1  OutDataTypeStr=fixdt(0, floor(36/voteWL), 0)  SampleTime=-1
  Simple Hough Accumulator : Subsystem
  Switch : Switch  Criteria=u2 > Threshold
  Switch1 : Switch  Criteria=u2 > Threshold
  Switch3 : Switch  Criteria=u2 > Threshold
  Terminator : Terminator
  ThetaMax : Constant  Value=Ntheta/floor(36/voteWL)-1  OutDataTypeStr=uint32  SampleTime=-1
  Pixel : Outport  VectorParamsAs1DForOutWhenUnconnected=off
  last_out : Outport  Port=2  VectorParamsAs1DForOutWhenUnconnected=off
  valid_out : Outport  Port=3  VectorParamsAs1DForOutWhenUnconnected=off
  user_out : Outport  Port=4  VectorParamsAs1DForOutWhenUnconnected=off
  wires:
  Ready/1 -> Accumulator Control/5(ready)
  Constant/1 -> Simple Hough Accumulator/1(Zero)
  Constant1/1 -> Simple Hough Accumulator/2(Vote)
  Switch/1 -> Simple Hough Accumulator/6(Polar)
  Accumulator Control/8(hEnd) -> last_out/1
  Accumulator Control/9(vStart) -> user_out/1
  Accumulator Control/11(valid) -> valid_out/1
  Accumulator Control/4(sel) -> Switch/2, Switch3/2, Switch1/2, Simple Hough Accumulator/7(Sel)
  Switch1/1 -> Simple Hough Accumulator/5(Edge)
  Accumulator Control/6(idx) -> Delay2/1
  Threshold/1 -> Simple Hough Accumulator/3(Thresh)
  Accumulator Control/5(read) -> Simple Hough Accumulator/8(Read)
  RhoMax/1 -> Accumulator Control/6(rhomax)
  ThetaMax/1 -> Accumulator Control/7(thetamax)
  Constant2/1 -> Accumulator Control/4(mode)
  Rho/1 -> Switch/1
  Accumulator Control/3(address) -> Data Type Conversion/1
  Output Generation/1(" Pixel") -> Pixel/1
  Delay2/1 -> Output Generation/2("idx ")
  Accumulator Control/2(clear) -> Switch1/3
  Data Type Conversion/1 -> Switch/3
  Accumulator Control/12(debug_state) -> Terminator/1
  Shift/1 -> Switch3/1
  ShiftMax/1 -> Accumulator Control/8(shiftmax)
  Accumulator Control/1(shift) -> Gain/1
  Switch3/1 -> Simple Hough Accumulator/4(Shift)
  Gain/1 -> Switch3/3
  Simple Hough Accumulator/1(vHPS) -> Output Generation/1("vHPS ")
  vEdge/1 -> Switch1/1
  valid_in/1 -> Accumulator Control/3(fvalid)
  user_in/1 -> HDL Counter/1, Accumulator Control/1(sof)
  HDL Counter/1 -> Compare To Constant3/1
  Compare To Constant3/1 -> Accumulator Control/2(eof)
  last_in/1 -> HDL Counter/2

== system hybrid_lht_accumulator_backup/Hybrid LHT2/Hybrid LHT Kernel ==
  s_axis_tvalid : Inport
  s_axis_tdata : Inport  Port=2
  s_axis_tuser : Inport  Port=3
  s_axis_tlast : Inport  Port=4
  AND : Logic  IconShape=distinctive  AllPortsSameDT=off  OutDataTypeStr=boolean
  Edge Slice : hdlsllib/Logic and Bit Operations/Bit Slice  lidx=ceil(log2(round(theta(end)/dTheta)+1))  ridx=ceil(log2(round(theta(end)/dTheta)+1))
      settings: SourceProductName=Simulink  SourceProductBaseCode=SL
  Extract Active Votes : Subsystem
  Gradient Kernel System : Subsystem
  Selector1 : Selector  NumberOfDimensions=2  IndexMode=Zero-based  InputPortWidth=3  IndexOptions=Index vector (dialog),Index vector (port)  Indices=0,1  OutputSizes=1,1
  Selector6 : Selector  NumberOfDimensions=2  IndexMode=Zero-based  InputPortWidth=3  IndexOptions=Index vector (dialog),Index vector (port)  Indices=0,1  OutputSizes=1,1
  Theta Slice : hdlsllib/Logic and Bit Operations/Bit Slice  lidx=ceil(log2(round(theta(end)/dTheta)+1))-1  ridx=0
      settings: SourceProductName=Simulink  SourceProductBaseCode=SL
  X Counter : hdlsllib/Sources/HDL Counter  CountType=Count limited  CountInit=-width/2  CountStep=1  CountMax=width/2-1  CountFromType=Initial value  CountFrom=-width/2  CountResetPort=off  CountLoadPort=off  CountEnbPort=on  CountDirPort=off  CountDataType=Signed  CountWordLen=ceil(log2(width))  CountFracLen=0  CountSampTime=1
      settings: SourceProductName=Simulink
  Y Counter : hdlsllib/Sources/HDL Counter  CountType=Count limited  CountInit=-height/2  CountStep=1  CountMax=height/2-1  CountFromType=Initial value  CountFrom=-height/2  CountResetPort=off  CountLoadPort=off  CountEnbPort=on  CountDirPort=off  CountDataType=Signed  CountWordLen=ceil(log2(height))  CountFracLen=0  CountSampTime=1
      settings: SourceProductName=Simulink
  m_axis_tvalid : Outport
  m_axis_tuser : Outport  Port=2
  m_axis_tlast : Outport  Port=3
  hough_param : Outport  Port=4
  edge : Outport  Port=5
  shift : Outport  Port=6
  wires:
  Y Counter/1 -> Gradient Kernel System/3(Y)
  X Counter/1 -> Gradient Kernel System/2(X)
  s_axis_tdata/1 -> Theta Slice/1, Edge Slice/1
  AND/1 -> Y Counter/1
  Gradient Kernel System/1(vEdge) -> edge/1
  Gradient Kernel System/3(Shift) -> Selector1/1
  Gradient Kernel System/2(Rho) -> Selector6/1
  Extract Active Votes/1(Index) -> Selector1/2, Selector6/2
  Selector6/1 -> hough_param/1
  Selector1/1 -> shift/1
  Edge Slice/1 -> Gradient Kernel System/1(Edge)
  Theta Slice/1 -> Extract Active Votes/1(Theta), Gradient Kernel System/4(Theta)
  s_axis_tuser/1 -> m_axis_tuser/1
  s_axis_tlast/1 -> m_axis_tlast/1, AND/2
  s_axis_tvalid/1 -> m_axis_tvalid/1, X Counter/1, AND/1

== system hybrid_lht_accumulator_backup/Hybrid LHT2/Hybrid LHT Kernel1 ==
  s_axis_tvalid : Inport
  s_axis_tdata : Inport  Port=2
  s_axis_tuser : Inport  Port=3
  s_axis_tlast : Inport  Port=4
  AND : Logic  IconShape=distinctive  AllPortsSameDT=off  OutDataTypeStr=boolean
  Edge Slice : hdlsllib/Logic and Bit Operations/Bit Slice  lidx=ceil(log2(round(theta(end)/dTheta)+1))  ridx=ceil(log2(round(theta(end)/dTheta)+1))
      settings: SourceProductName=Simulink  SourceProductBaseCode=SL
  Gradient Kernel System : Subsystem
  Selector : Selector  NumberOfDimensions=2  IndexMode=Zero-based  InputPortWidth=3  IndexOptions=Index vector (dialog),Index vector (dialog)  Indices=0,0  OutputSizes=1,1
  Selector1 : Selector  NumberOfDimensions=2  IndexMode=Zero-based  InputPortWidth=3  IndexOptions=Index vector (dialog),Index vector (dialog)  Indices=0,0  OutputSizes=1,1
  Terminator : Terminator
  Terminator1 : Terminator
  Theta Slice : hdlsllib/Logic and Bit Operations/Bit Slice  lidx=ceil(log2(round(theta(end)/dTheta)+1))-1  ridx=0
      settings: SourceProductName=Simulink  SourceProductBaseCode=SL
  X Counter : hdlsllib/Sources/HDL Counter  CountType=Count limited  CountInit=-width/2  CountStep=1  CountMax=width/2-1  CountFromType=Initial value  CountFrom=-width/2  CountResetPort=off  CountLoadPort=off  CountEnbPort=on  CountDirPort=off  CountDataType=Signed  CountWordLen=ceil(log2(width))  CountFracLen=0  CountSampTime=1
      settings: SourceProductName=Simulink
  Y Counter : hdlsllib/Sources/HDL Counter  CountType=Count limited  CountInit=-height/2  CountStep=1  CountMax=height/2-1  CountFromType=Initial value  CountFrom=-height/2  CountResetPort=off  CountLoadPort=off  CountEnbPort=on  CountDirPort=off  CountDataType=Signed  CountWordLen=ceil(log2(height))  CountFracLen=0  CountSampTime=1
      settings: SourceProductName=Simulink
  m_axis_tvalid : Outport
  m_axis_tuser : Outport  Port=2
  m_axis_tlast : Outport  Port=3
  hough_param : Outport  Port=4
  edge : Outport  Port=5
  shift : Outport  Port=6
  wires:
  Selector1/1 -> Terminator1/1
  Selector/1 -> Terminator/1
  Gradient Kernel System/3(Shift) -> shift/1, Selector1/1
  Gradient Kernel System/1(vEdge) -> edge/1
  Gradient Kernel System/2(Rho) -> hough_param/1, Selector/1
  Edge Slice/1 -> Gradient Kernel System/1(Edge)
  Theta Slice/1 -> Gradient Kernel System/4(Theta)
  s_axis_tvalid/1 -> X Counter/1, AND/1, m_axis_tvalid/1
  AND/1 -> Y Counter/1
  s_axis_tlast/1 -> AND/2, m_axis_tlast/1
  s_axis_tdata/1 -> Edge Slice/1, Theta Slice/1
  s_axis_tuser/1 -> m_axis_tuser/1
  X Counter/1 -> Gradient Kernel System/2(X)
  Y Counter/1 -> Gradient Kernel System/3(Y)

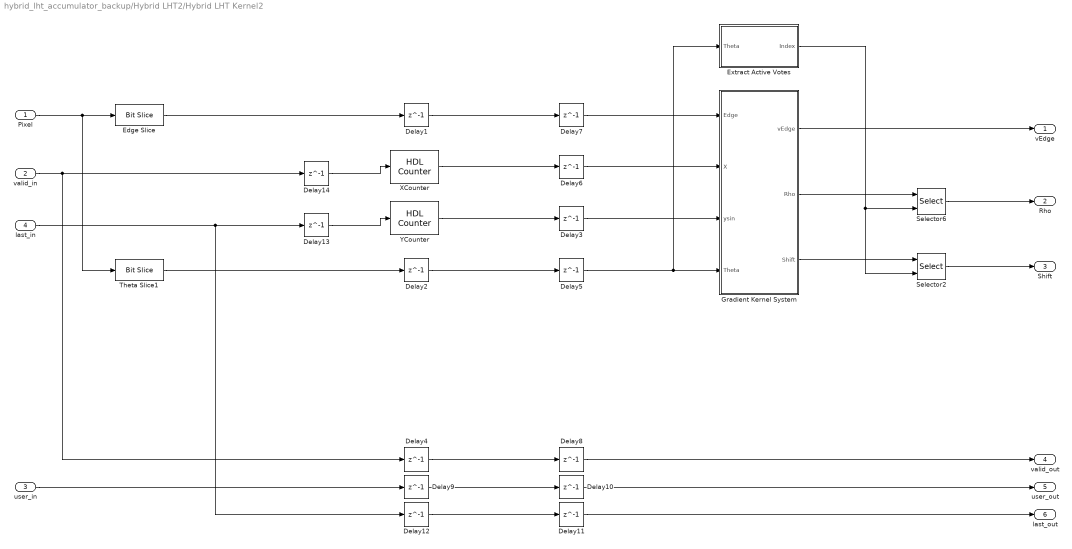
== system hybrid_lht_accumulator_backup/Hybrid LHT2/Hybrid LHT Kernel2 ==
  Pixel : Inport
  valid_in : Inport  Port=2
  user_in : Inport  Port=3
  last_in : Inport  Port=4
  Delay{1..14} (14 alike) : Delay  DelayLength=1
  Edge Slice : hdlsllib/Logic and Bit Operations/Bit Slice  lidx=8  ridx=8
  Extract Active Votes : Subsystem
  Gradient Kernel System : Subsystem
  Selector2 : Selector  NumberOfDimensions=2  IndexMode=Zero-based  InputPortWidth=3  IndexOptions=Index vector (dialog),Index vector (port)  Indices=0,1  OutputSizes=1,1
  Selector6 : Selector  NumberOfDimensions=2  IndexMode=Zero-based  InputPortWidth=3  IndexOptions=Index vector (dialog),Index vector (port)  Indices=0,1  OutputSizes=1,1
  Theta Slice1 : hdlsllib/Logic and Bit Operations/Bit Slice  lidx=7  ridx=0
  XCounter : hdlsllib/Sources/HDL Counter  CountType=Count limited  CountInit=-w/2  CountStep=1  CountMax=w/2-1  CountFromType=Initial value  CountFrom=-w/2  CountResetPort=off  CountLoadPort=off  CountEnbPort=on  CountDirPort=off  CountDataType=Signed  CountWordLen=ceil(log2(w/2))+1  CountFracLen=0  CountSampTime=1
      settings: SourceProductBaseCode=HD
  YCounter : hdlsllib/Sources/HDL Counter  CountType=Count limited  CountInit=-h/2  CountStep=1  CountMax=h/2-1  CountFromType=Initial value  CountFrom=-h/2  CountResetPort=off  CountLoadPort=off  CountEnbPort=on  CountDirPort=off  CountDataType=Signed  CountWordLen=ceil(log2(h/2))+1  CountFracLen=0  CountSampTime=1
      settings: SourceProductBaseCode=HD
  vEdge : Outport  VectorParamsAs1DForOutWhenUnconnected=off
  Rho : Outport  Port=2  VectorParamsAs1DForOutWhenUnconnected=off
  Shift : Outport  Port=3  VectorParamsAs1DForOutWhenUnconnected=off
  valid_out : Outport  Port=4  VectorParamsAs1DForOutWhenUnconnected=off
  user_out : Outport  Port=5  VectorParamsAs1DForOutWhenUnconnected=off
  last_out : Outport  Port=6  VectorParamsAs1DForOutWhenUnconnected=off
  wires:
  Selector6/1 -> Rho/1
  Selector2/1 -> Shift/1
  Extract Active Votes/1(Index) -> Selector2/2, Selector6/2
  Pixel/1 -> Theta Slice1/1, Edge Slice/1
  Gradient Kernel System/2(Rho) -> Selector6/1
  Gradient Kernel System/3(Shift) -> Selector2/1
  Gradient Kernel System/1(vEdge) -> vEdge/1
  Delay2/1 -> Delay5/1
  XCounter/1 -> Delay6/1
  Delay1/1 -> Delay7/1
  Delay4/1 -> Delay8/1
  Delay5/1 -> Extract Active Votes/1(Theta), Gradient Kernel System/4(Theta)
  Delay6/1 -> Gradient Kernel System/2(X)
  Delay7/1 -> Gradient Kernel System/1(Edge)
  Delay8/1 -> valid_out/1
  Edge Slice/1 -> Delay1/1
  Theta Slice1/1 -> Delay2/1
  YCounter/1 -> Delay3/1
  Delay3/1 -> Gradient Kernel System/3(ysin)
  valid_in/1 -> Delay4/1, Delay14/1
  Delay10/1 -> user_out/1
  Delay9/1 -> Delay10/1
  user_in/1 -> Delay9/1
  last_in/1 -> Delay12/1, Delay13/1
  Delay12/1 -> Delay11/1
  Delay11/1 -> last_out/1
  Delay13/1 -> YCounter/1
  Delay14/1 -> XCounter/1

== system hybrid_lht_accumulator_backup/Hybrid LHT/Hybrid LHT Accumulator/Output Generation ==
  "vHPS " : Inport
  "idx " : Inport  Port=2
  Backprojection : Subsystem  VariantControl=Backprojection
  HPS Readout : Subsystem  VariantControl=Passthrough
  " Pixel" : Outport  VectorParamsAs1DForOutWhenUnconnected=off

== system hybrid_lht_accumulator_backup/Hybrid LHT/Hybrid LHT Accumulator/Simple Hough Accumulator ==
  Zero : Inport
  Vote : Inport  Port=2
  Thresh : Inport  Port=3
  Shift : Inport  Port=4  Partition=on  PartitionDimension=2  PartitionWidth=1  PartitionOffset=0
  Edge : Inport  Port=5
  Polar : Inport  Port=6  Partition=on  PartitionDimension=2  PartitionWidth=1  PartitionOffset=0
  Sel : Inport  Port=7
  Read : Inport  Port=8
  Flag Generator : Subsystem  VariantControlMode=Label  Variant=on  VariantControl=Backprop  LabelModeActiveChoice=Passthrough
  For Each : ForEach  DisableCoverage=on
  Hough Accumulator : Subsystem
  Keep Flag : Subsystem  VariantControlMode=Label  Variant=on  VariantControl=Backprop  LabelModeActiveChoice=Passthrough
  Separate Bits : Subsystem  VariantControlMode=Label  Variant=on  VariantControl=Backprop  LabelModeActiveChoice=Passthrough
  vHPS : Outport  ConcatenationDimension=2  VectorParamsAs1DForOutWhenUnconnected=off
  wires:
  Hough Accumulator/2(HPS) -> vHPS/1, Separate Bits/1("VoteFlagIn ")
  Vote/1 -> Hough Accumulator/3(Vote)
  Sel/1 -> Hough Accumulator/5(Sel)
  Polar/1 -> Hough Accumulator/6(Rho)
  Edge/1 -> Hough Accumulator/7(Edge)
  Separate Bits/2(" VoteOut") -> Hough Accumulator/8(FromFlag), Flag Generator/1("ReadOut ")
  Thresh/1 -> Flag Generator/2("Thresh ")
  Zero/1 -> Flag Generator/3("ZeroData ")
  Read/1 -> Flag Generator/4("ReadValid ")
  Flag Generator/1(" ZeroDataFlagged") -> Hough Accumulator/2(Zero)
  Separate Bits/1(" FlagOut") -> Keep Flag/1("FlagIn ")
  Hough Accumulator/1(ToFlag) -> Keep Flag/2("VoteIn ")
  Keep Flag/1(" VoteFlagOut") -> Hough Accumulator/1(Data)
  Shift/1 -> Hough Accumulator/4(Shift)
